simulink model "simulation"  (R2022b)
settings: Solver=VariableStepAuto  StartTime=0.0  StopTime=10.0  RelTol=1e-3
values from neighbouring files (symbols this model uses):
  a = -1/tau    (= -50)    [data_modele.m]
  b = context.isCodeGenTarget('rtw')    [DCMotor1Set.m]    (also in DCMotor2Set.m; Enc1Period.m; Enc1Read.m; data_modele.m = 2500)
  k1 = K(1, 2)    [data_modele.m]
  k2 = K(1, 1)    [data_modele.m]
undefined symbols (not defined in the file or in its folder): sigbuilder_block
libraries: eeLuenbergerObserver x1
settings Model: Creator=mtroislo  LastModifiedBy=mtroislo

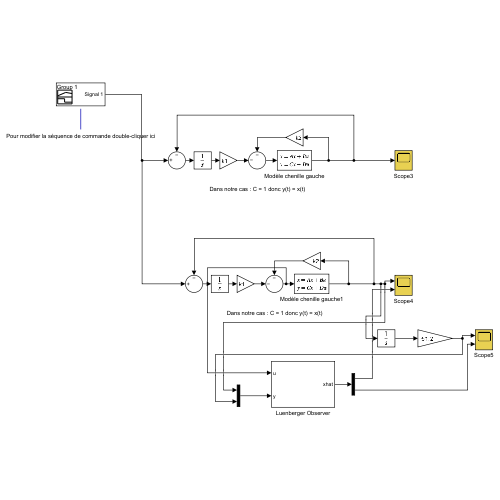
[thumbnail: Simulink's stored preview of the top-level diagram]
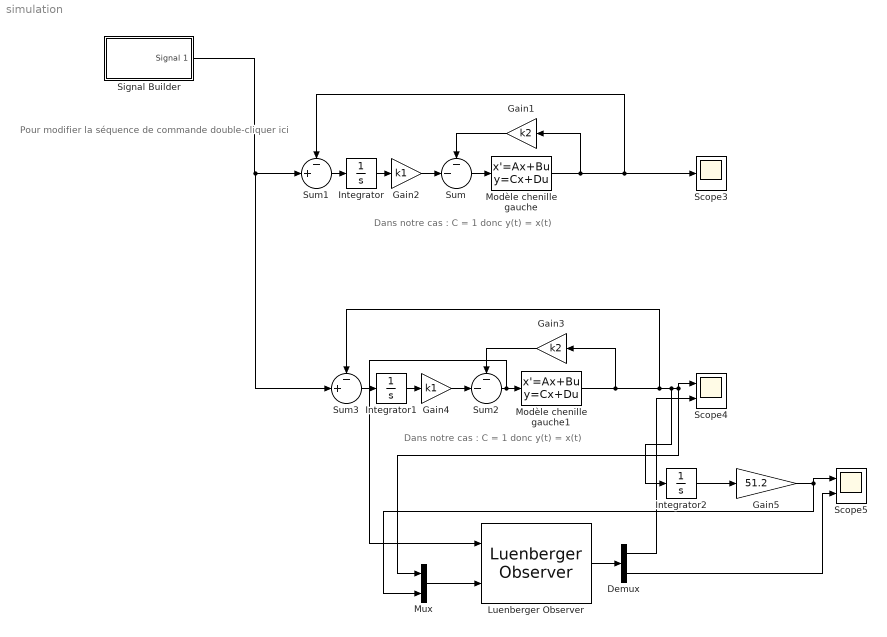
== system simulation ==
  note: Pour modifier la séquence de commande double-cliquer ici
  note: Dans notre cas : C = 1 donc y(t) = x(t)
  note: Dans notre cas : C = 1 donc y(t) = x(t)
  Demux : Demux  Outputs=2
  Gain1 : Gain  Gain=k2
  Gain2 : Gain  Gain=k1
  Gain3 : Gain  Gain=k2
  Gain4 : Gain  Gain=k1
  Gain5 : Gain  Gain=51.2
  Integrator : Integrator
  Integrator1 : Integrator
  Integrator2 : Integrator
  Luenberger Observer : eeLuenbergerObserver/Luenberger Observer  StateSpaceType=Discrete-time  Ad=1  Bd=1  Cd=1  Dd=1  A=1  B=1  C=1  D=1  ObserverDesign=Desired eigenvalues  Ld=1  DesiredEigenvalues=0  x0=0  Tsd=0.1  Ts=0.1
      settings: LibrarySourceBlock=ee_sl_lib/Observers/Luenberger Observer
  Modèle chenille gauche : StateSpace  A=a  B=b  D=0  InitialCondition=0
  Modèle chenille gauche1 : StateSpace  A=a  B=b  D=0  InitialCondition=0
  Mux : Mux  Inputs=2
  Scope3 : Scope
  Scope4 : Scope  NumInputPorts=2
  Scope5 : Scope  NumInputPorts=2
  Signal Builder : Subsystem  Tag=STV Subsys  LoadFcn=sigbuilder_block('load');  StartFcn=sigbuilder_block('start');  StopFcn=sigbuilder_block('stop');  ClipboardFcn=sigbuilder_block('clipboard');  mask(Sigbuilder block){tuvar=[0:10]}
      mask help: Simulink:masks:SigbuilderBlock_MD
      mask init:
      | if ~strcmp(get_param(bdroot(gcbh),'SimulationStatus'),'stopped') tuvar = sigbuilder_block('maskInit'); end
      settings: CopyFcn=sigbuilder_block('copy');  DeleteFcn=sigbuilder_block('delete');  ModelCloseFcn=sigbuilder_block('modelClose');  PreSaveFcn=sigbuilder_block('preSave');  PauseFcn=sigbuilder_block('pause');  ContinueFcn=sigbuilder_block('continue');  NameChangeFcn=sigbuilder_block('namechange');  OpenFcn=sigbuilder_block('open',[382.125 217.125 550.5 400.5 ]);  CloseFcn=sigbuilder_block('close');
      mask Display: plot(0, 0, 100, 100,[2, 2, 32, 32, 2], [68, 8, 8, 68, 68],[32, 2], [38, 38], [32, 19, 2],[53, 60, 44], [32, 17, 17, 2],[16, 16, 31, 31]);txt = getActiveGroup(gcbh);text(2, 100, txt,'verticalAlignment', 'top');
  Sum : Sum  Inputs=--|
  Sum1 : Sum  Inputs=-+|
  Sum2 : Sum  Inputs=--|
  Sum3 : Sum  Inputs=-+|
  wires:
  Demux/1 -> Scope4/2
  Demux/2 -> Scope5/2
  Integrator2/1 -> Gain5/1
  Gain5/1 -> Mux/2, Scope5/1
  Mux/1 -> Luenberger Observer/2
  Modèle chenille gauche1/1 -> Integrator2/1, Mux/1, Scope4/1, Sum3/1, Gain3/1
  Gain3/1 -> Sum2/1
  Luenberger Observer/1 -> Demux/1
  Gain1/1 -> Sum/1
  Modèle chenille gauche/1 -> Scope3/1, Sum1/1, Gain1/1
  Gain2/1 -> Sum/2
  Sum/1 -> Modèle chenille gauche/1
  Integrator/1 -> Gain2/1
  Sum1/1 -> Integrator/1
  Signal Builder/1(Signal 1) -> Sum3/2, Sum1/2
  Sum3/1 -> Integrator1/1
  Sum2/1 -> Luenberger Observer/1, Modèle chenille gauche1/1
  Integrator1/1 -> Gain4/1
  Gain4/1 -> Sum2/2

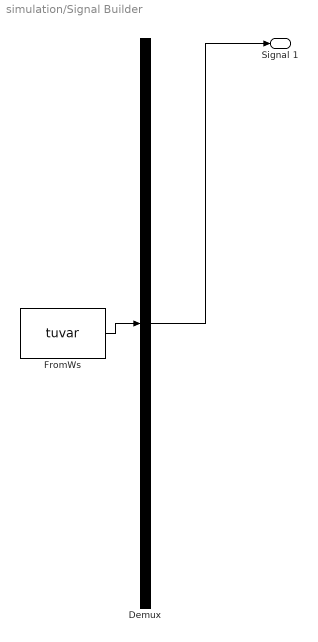
== system simulation/Signal Builder ==
  Demux : Demux  Tag=STV Demux  Outputs=1
      settings: DisplayOption=none
  FromWs : FromWorkspace  Tag=STV FromWs  VariableName=tuvar
      SigBuilderData=|
      | common.afterFinalStr = 'Extrapolate'
      | common.sampleTime = 0
      | dataSet.timeRange = [0 10]
      | dataSet.name = 'Group 1'
      | sbobj.Groups.Name = 'Group 1'
      | sbobj.Groups.Signals.Name = 'Signal 1'
      | sbobj.Groups.Signals.XData = [0 1 1 1.5 1.5 4 4 5 5 7 7 8 8 9 9 9.5 9.5 10]
      | sbobj.Groups.Signals.YData = [0 0 7 7 0 0 4 4 0 0 -4 -4 0 0 -7 -7 0 0]
  Signal 1 : Outport  Tag=STV Outport  VectorParamsAs1DForOutWhenUnconnected=off
  wires:
  Demux/1 -> Signal 1/1
  FromWs/1 -> Demux/1
